simulink model "HVDC_Model"  (R2024a)
settings: Solver=VariableStepAuto  StartTime=0.0  StopTime=10.0  RelTol=1e-3
undefined symbols (not defined in the file or in its folder): D1, Delta, Fnom_I, Fnom_R, Idc_nom, lagging, pulse, Ts, Vdc_nom, VLL_nom_I, VLL_nom_R
libraries: spsThreePhaseHarmonicFilterLib x6, spsUniversalBridgeLib x4, spsGroundLib x3, spsPulseGeneratorThyristor12PulseLib x3, spsVoltageMeasurementLib x3, spsThreePhaseSourceLib x2, spsThreePhaseParallelRLCBranchLib x2, spsThreePhaseSeriesRLCLoadLib x2, spsPLL3phLib x2, spsThreePhaseTransformerThreeWindingsLib x2, spsCurrentMeasurementLib x2, spsSeriesRLCBranchLib x1
settings Model: Creator=E370_  LastModifiedBy=E370_

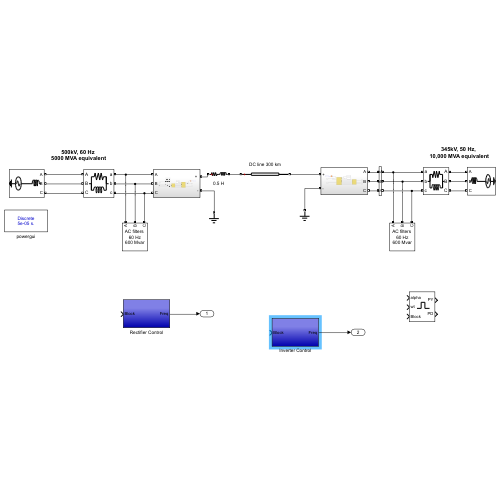
[thumbnail: Simulink's stored preview of the top-level diagram]
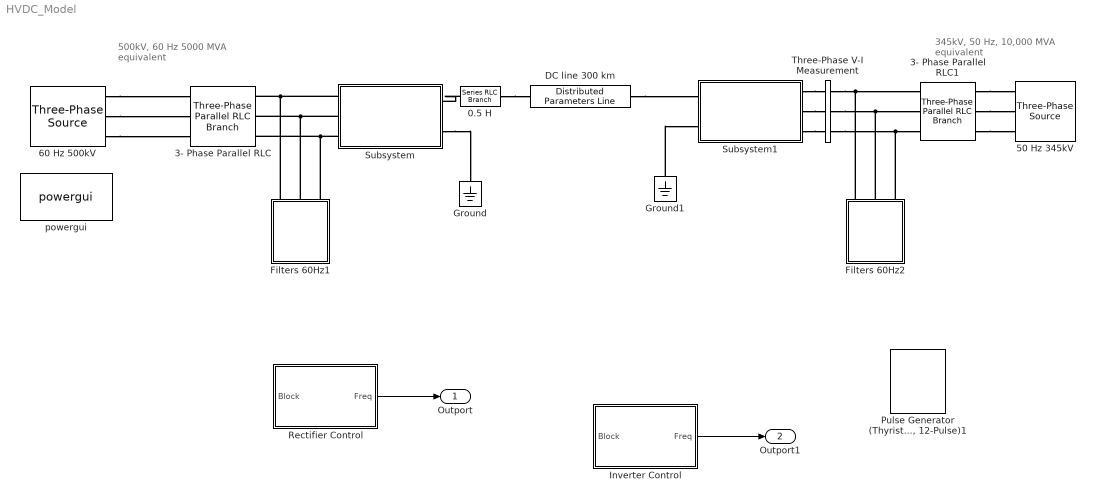
== system HVDC_Model ==
  note: 500kV, 60 Hz
      |  5000 MVA equivalent
  note: 345kV, 50 Hz,
      | 10,000 MVA equivalent
  " 50 Hz 345kV  " : spsThreePhaseSourceLib/Three-Phase Source  InternalConnection=Yg  VoltagePhases=off  Voltage=VLL_nom_I  PhaseAngle=0  Voltage_phases=[25e3 25e3 25e3]/sqrt(3)  PhaseAngles_phases=[0 -120 +120]  Frequency=Fnom_I  NonIdealSource=on  SpecifyImpedance=off  Resistance=0  Inductance=28.0e-3  ShortCircuitLevel=0  BaseVoltage=0  XRratio=0  BusType=swing  Pref=0  Qref=0  Prefabc=[10e3, 10e3, 10e3]  Qrefabc=[0, 0, 0]  Qmin=-inf  Qmax=inf
  " 60 Hz 500kV" : spsThreePhaseSourceLib/Three-Phase Source  InternalConnection=Yg  VoltagePhases=off  Voltage=VLL_nom_R  PhaseAngle=0  Voltage_phases=[25e3 25e3 25e3]/sqrt(3)  PhaseAngles_phases=[0 -120 +120]  Frequency=Fnom_R  NonIdealSource=on  SpecifyImpedance=off  Resistance=0  Inductance=98.03e-3  ShortCircuitLevel=0  BaseVoltage=0  XRratio=0  BusType=swing  Pref=0  Qref=0  Prefabc=[10e3, 10e3, 10e3]  Qrefabc=[0, 0, 0]  Qmin=-inf  Qmax=inf
  0.5 H : spsSeriesRLCBranchLib/Series RLC Branch  LConnTagsString=__new0  RConnTagsString=__new0  BranchType=RL  Resistance=1  Inductance=0.5  SetiL0=off  InitialCurrent=0  Capacitance=1.0  Setx0=off  InitialVoltage=0  Measurements=None
  3- Phase Parallel RLC : spsThreePhaseParallelRLCBranchLib/Three-Phase Parallel RLC Branch  LConnTagsString=A|B|C  RConnTagsString=A|B|C  BranchType=RL  Resistance=26.07  Inductance=48.86e-3  Capacitance=1.0  Measurements=None
  3- Phase Parallel RLC1 : spsThreePhaseParallelRLCBranchLib/Three-Phase Parallel RLC Branch  LConnTagsString=A|B|C  RConnTagsString=A|B|C  BranchType=RL  Resistance=6.205  Inductance=13.96e-3  Capacitance=1.0  Measurements=None
  DC line 300 km : spsDistributedParametersLineLib/Distributed Parameters Line  Phases=1  Length=300  Frequency=60  Resistance=0.015  Inductance=0.792e-3  Capacitance=14.4e-9  x1=[-0.00105 -6.18058111349283e-12;-0.001 -6.09272096015694e-12;-0.00095 -6.00369609044989e-12;-0.0009 -5.91353789360421e-12;-0.00085 -5.82227791484294e-12;-0.0008 -5.7299478442921e-12;-0.00075 -5.63657950590245e-12;-0.0007 -5.54220484638449e-12;-0.00065 -5.44685592416066e-12;-0.0006 -5.35056489833836e-12;-0.00055 -5.2533640177079e-12;-0.0005 -5.15528560976897e-12;-0.00045 -5.05636206978949e-12;-0.0004 -4.95662584990061e-12;-0.00035 -4.85610944823157e-12;-0.0003 -4.75484539808807e-12;-0.00025 -4.65286625717792e-12;-0.0002 -4.55020459688746e-12;-0.00015 -4.44689299161251e-12;-0.0001 -4.34296400814731e-12;-5e-05 -4.23845019513496e-12]  x2=[-0.00105 -5.4796147498648e-12;-0.001 -5.38394831103393e-12;-0.00095 -5.28731700560248e-12;-0.0009 -5.18975488737601e-12;-0.00085 -5.09129610703133e-12;-0.0008 -4.99197490010943e-12;-0.00075 -4.89182557503596e-12;-0.0007 -4.79088250117334e-12;-0.00065 -4.68918009690885e-12;-0.0006 -4.58675281778278e-12;-0.00055 -4.48363514466077e-12;-0.0005 -4.37986157195443e-12;-0.00045 -4.27546659589437e-12;-0.0004 -4.17048470285956e-12;-0.00035 -4.06495035776722e-12;-0.0003 -3.95889799252695e-12;-0.00025 -3.85236199456322e-12;-0.0002 -3.74537669541008e-12;-0.00015 -3.63797635938187e-12;-0.0001 -3.53019517232379e-12;-5e-05 -3.42206723044614e-12]  x3=[-0.00105 -3.41290835471429e-14;-0.001 -3.36568958149302e-14;-0.00095 -3.31769543764507e-14;-0.0009 -3.26894283733644e-14;-0.00085 -3.21944886050515e-14;-0.0008 -3.16923074685244e-14;-0.00075 -3.11830588980277e-14;-0.0007 -3.06669183043476e-14;-0.00065 -3.0144062513852e-14;-0.0006 -2.96146697072825e-14;-0.00055 -2.90789193583197e-14;-0.0005 -2.85369921719432e-14;-0.00045 -2.79890700226075e-14;-0.0004 -2.74353358922559e-14;-0.00035 -2.68759738081922e-14;-0.0003 -2.63111687808334e-14;-0.00025 -2.57411067413637e-14;-0.0002 -2.5165974479311e-14;-0.00015 -2.45859595800679e-14;-0.0001 -2.40012503623781e-14;-5e-05 -2.34120358158086e-14]  x4=[-0.00105 -2.27784758684538e-14;-0.001 -2.25723505250607e-14;-0.00095 -2.23621997542686e-14;-0.0009 -2.21481181558178e-14;-0.00085 -2.1930200735571e-14;-0.0008 -2.17085428670839e-14;-0.00075 -2.14832402532907e-14;-0.0007 -2.12543888883198e-14;-0.00065 -2.10220850194532e-14;-0.0006 -2.07864251092444e-14;-0.00055 -2.05475057978099e-14;-0.0005 -2.0305423865308e-14;-0.00045 -2.00602761946182e-14;-0.0004 -1.98121597342372e-14;-0.00035 -1.9561171461403e-14;-0.0003 -1.9307408345463e-14;-0.00025 -1.90509673114976e-14;-0.0002 -1.87919452042148e-14;-0.00015 -1.85304387521266e-14;-0.0001 -1.82665445320231e-14;-5e-05 -1.80003589337544e-14]  x5=0.00101312980412186  V1=ones(3,3)  V2=ones(3,3)  I1=ones(3,3)  I2=ones(3,3)  nHarmo=1  Measurements=Phase-to-ground voltages  Decoupling=off  VsMag0=0  VrMag0=0  VsAngle0=0  VrAngle0=0  IsMag0=0  IrMag0=0  IsAngle0=0  IrAngle0=0
      settings: AttributesFormatString=\n
  Filters 60Hz1 : Subsystem
      mask Display: disp('AC filters \n60 Hz\n600 Mvar')
  Filters 60Hz2 : Subsystem
      mask Display: disp('AC filters \n60 Hz\n600 Mvar')
  Ground : spsGroundLib/Ground  LConnTagsString=a
  Ground1 : spsGroundLib/Ground  LConnTagsString=a
  Inverter Control : Subsystem
  "Pulse Generator (Thyristor, 12-Pulse)1" : spsPulseGeneratorThyristor12PulseLib/Pulse Generator (Thyristor, 12-Pulse)  GenType=12-pulse  Delta=D1 (lagging)  pwidth=60  Double_Pulse=off  Ts=0
      settings: LibrarySourceBlock=|
      | sps_lib/Power Electronics/Power Electronics Control/Pulse Generator
      | (Thyristor, 12-Pulse)
  Rectifier Control : Subsystem
  Subsystem : Subsystem
  Subsystem1 : Subsystem
  Three-Phase V-I Measurement : spsThreePhaseVIMeasurementLib/Three-Phase V-I Measurement  VoltageMeasurement=phase-to-ground  SetLabelV=on  LabelV=Vabc_I  Vpu=on  VpuLL=off  CurrentMeasurement=yes  SetLabelI=on  LabelI=Iabc_I  Ipu=on  Pbase=100e6  Vbase=345e3  OutputType=Complex  PhasorSimulation=off  PSBequivalent=0
  powergui : spspowerguiLib/powergui  Priority=2  SimulationMode=Discrete  SampleTime=Ts  frequency=60  Iterations=50  frequencyindice=60  Pbase=100e6  ErrMax=1e-4  UnitsV=kV  UnitsW=MW  buscounter=0  FunctionMessages=off  echomessages=off  EnableUseOfTLC=off  CurrentSourceSwitches=off  DisableSnubberDevices=off  DisableRonSwitches=off  DisableVfSwitches=off  DisplayEquations=off  AutomaticDiscreteSolvers=off  SolverType=Tustin  Interpol=off  ExternalGateDelay=off  methode=off  Ts=0  x0status=blocks  SPID=off  SwTol=0  HookPort=off  NonlinearTolerance=1e-4  nMaxIteration=100  ContinueOnMaxIteration=off  RestoreLinks=warning  ResistiveCurrentMeasurement=off  Frange=[10:2:1500]  Ylog=off  Xlog=off  ShowGrid=off  save=off  variable=ZData  structure=0  ZoomFFT=on  StartTime=0.0  cycles=1  DisplayStyle=off  fundamental=60  FreqAxis=off  MaxFrequency=1000  frequencyindicesteady=1  RmsSteady=1  display=off
  Outport : Outport
  Outport1 : Outport  Port=2
  wires:
  Rectifier Control/1(Freq) -> Outport/1
  Inverter Control/1(Freq) -> Outport1/1
  connections:
  Subsystem/RConn2 -- Ground/LConn1
  " 60 Hz 500kV"/RConn1 -- 3- Phase Parallel RLC/LConn1
  " 60 Hz 500kV"/RConn3 -- 3- Phase Parallel RLC/LConn3
  " 60 Hz 500kV"/RConn2 -- 3- Phase Parallel RLC/LConn2
  Subsystem/LConn3 -- 3- Phase Parallel RLC/RConn3 -- Filters 60Hz1/LConn3
  Subsystem/LConn2 -- 3- Phase Parallel RLC/RConn2 -- Filters 60Hz1/LConn2
  Subsystem/LConn1 -- 3- Phase Parallel RLC/RConn1 -- Filters 60Hz1/LConn1
  3- Phase Parallel RLC1/LConn1 -- " 50 Hz 345kV  "/RConn1
  3- Phase Parallel RLC1/LConn2 -- " 50 Hz 345kV  "/RConn2
  3- Phase Parallel RLC1/LConn3 -- " 50 Hz 345kV  "/RConn3
  Filters 60Hz2/LConn1 -- 3- Phase Parallel RLC1/RConn1 -- Three-Phase V-I Measurement/RConn1
  Filters 60Hz2/LConn2 -- 3- Phase Parallel RLC1/RConn2 -- Three-Phase V-I Measurement/RConn2
  Filters 60Hz2/LConn3 -- 3- Phase Parallel RLC1/RConn3 -- Three-Phase V-I Measurement/RConn3
  0.5 H/LConn1 -- Subsystem/RConn1
  0.5 H/RConn1 -- DC line 300 km/LConn1
  DC line 300 km/RConn1 -- Subsystem1/RConn1
  Ground1/LConn1 -- Subsystem1/RConn2
  Subsystem1/LConn1 -- Three-Phase V-I Measurement/LConn1
  Subsystem1/LConn2 -- Three-Phase V-I Measurement/LConn2
  Subsystem1/LConn3 -- Three-Phase V-I Measurement/LConn3

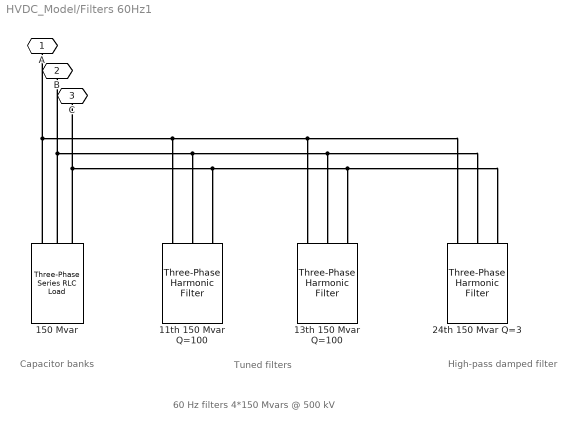
== system HVDC_Model/Filters 60Hz1 ==
  note: Capacitor banks
  note: Tuned filters
  note: High-pass
      | damped filter
  note: 60 Hz filters 4*150 Mvars @ 500 kV
  11th 150 Mvar Q=100 : spsThreePhaseHarmonicFilterLib/Three-Phase Harmonic Filter  LConnTagsString=A|B|C  FilterType=Single-tuned  FilterConnection=Y (grounded)  ParNom=[VLL_nom_R, Fnom_R]  Qc=0.25*(Vdc_nom*Idc_nom*0.6)  Fr=[11*Fnom_R]  Frd=[11*60 13*60]  Q=100  Measurements=None
      settings: AttributesFormatString=\n
  "13th 150 Mvar Q=100 " : spsThreePhaseHarmonicFilterLib/Three-Phase Harmonic Filter  LConnTagsString=A|B|C  FilterType=Single-tuned  FilterConnection=Y (grounded)  ParNom=[VLL_nom_R, Fnom_R]  Qc=0.25*(Vdc_nom*Idc_nom*0.6)  Fr=[13*Fnom_R]  Frd=[11*60 13*60]  Q=100  Measurements=None
      settings: AttributesFormatString=\n
  150 Mvar : spsThreePhaseSeriesRLCLoadLib/Three-Phase Series RLC Load  LConnTagsString=A|B|C  Configuration=Y (grounded)  NominalVoltage=VLL_nom_R  Vabc=[1e3 1e3 1e3]  Vabcp=[1e3 1e3 1e3]  NominalFrequency=Fnom_R  UnbalancedPower=off  ActivePower=0  InductivePower=0  CapacitivePower=0.25*(Vdc_nom*Idc_nom*0.6)  Pabc=[10e3 9e3 11e3]  QLabc=[100 90 110]  QCabc=[100 90 110]  Pabcp=[10e3 9e3 11e3]  QLabcp=[100 90 110]  QCabcp=[100 90 110]  Measurements=None  LoadType=constant Z
  24th 150 Mvar Q=3 : spsThreePhaseHarmonicFilterLib/Three-Phase Harmonic Filter  LConnTagsString=A|B|C  FilterType=High-pass  FilterConnection=Y (grounded)  ParNom=[VLL_nom_R, Fnom_R]  Qc=0.25*(Vdc_nom*Idc_nom*0.6)  Fr=[24*Fnom_R]  Frd=[11*60 13*60]  Q=3  Measurements=None
      settings: AttributesFormatString=\n
  A : PMIOPort  Side=Left
  B : PMIOPort  Port=2  Side=Left
  C : PMIOPort  Port=3  Side=Left
  connections:
  150 Mvar/LConn3 -- 24th 150 Mvar Q=3/LConn3 -- "13th 150 Mvar Q=100 "/LConn3 -- 11th 150 Mvar Q=100/LConn3 -- C/RConn1
  150 Mvar/LConn2 -- 24th 150 Mvar Q=3/LConn2 -- "13th 150 Mvar Q=100 "/LConn2 -- 11th 150 Mvar Q=100/LConn2 -- B/RConn1
  150 Mvar/LConn1 -- 24th 150 Mvar Q=3/LConn1 -- "13th 150 Mvar Q=100 "/LConn1 -- 11th 150 Mvar Q=100/LConn1 -- A/RConn1

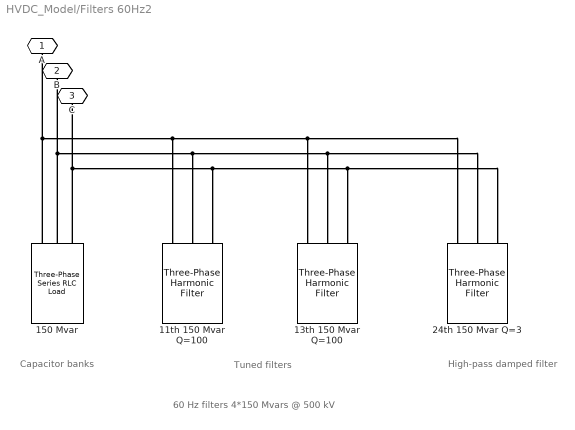
== system HVDC_Model/Filters 60Hz2 ==
  note: Capacitor banks
  note: Tuned filters
  note: High-pass
      | damped filter
  note: 60 Hz filters 4*150 Mvars @ 500 kV
  11th 150 Mvar Q=100 : spsThreePhaseHarmonicFilterLib/Three-Phase Harmonic Filter  LConnTagsString=A|B|C  FilterType=Single-tuned  FilterConnection=Y (grounded)  ParNom=[VLL_nom_R, Fnom_R]  Qc=0.25*(Vdc_nom*Idc_nom*0.6)  Fr=[11*Fnom_R]  Frd=[11*60 13*60]  Q=100  Measurements=None
      settings: AttributesFormatString=\n
  "13th 150 Mvar Q=100 " : spsThreePhaseHarmonicFilterLib/Three-Phase Harmonic Filter  LConnTagsString=A|B|C  FilterType=Single-tuned  FilterConnection=Y (grounded)  ParNom=[VLL_nom_R, Fnom_R]  Qc=0.25*(Vdc_nom*Idc_nom*0.6)  Fr=[13*Fnom_R]  Frd=[11*60 13*60]  Q=100  Measurements=None
      settings: AttributesFormatString=\n
  150 Mvar : spsThreePhaseSeriesRLCLoadLib/Three-Phase Series RLC Load  LConnTagsString=A|B|C  Configuration=Y (grounded)  NominalVoltage=VLL_nom_R  Vabc=[1e3 1e3 1e3]  Vabcp=[1e3 1e3 1e3]  NominalFrequency=Fnom_R  UnbalancedPower=off  ActivePower=0  InductivePower=0  CapacitivePower=0.25*(Vdc_nom*Idc_nom*0.6)  Pabc=[10e3 9e3 11e3]  QLabc=[100 90 110]  QCabc=[100 90 110]  Pabcp=[10e3 9e3 11e3]  QLabcp=[100 90 110]  QCabcp=[100 90 110]  Measurements=None  LoadType=constant Z
  24th 150 Mvar Q=3 : spsThreePhaseHarmonicFilterLib/Three-Phase Harmonic Filter  LConnTagsString=A|B|C  FilterType=High-pass  FilterConnection=Y (grounded)  ParNom=[VLL_nom_R, Fnom_R]  Qc=0.25*(Vdc_nom*Idc_nom*0.6)  Fr=[24*Fnom_R]  Frd=[11*60 13*60]  Q=3  Measurements=None
      settings: AttributesFormatString=\n
  A : PMIOPort  Side=Left
  B : PMIOPort  Port=2  Side=Left
  C : PMIOPort  Port=3  Side=Left
  connections:
  150 Mvar/LConn3 -- 24th 150 Mvar Q=3/LConn3 -- "13th 150 Mvar Q=100 "/LConn3 -- 11th 150 Mvar Q=100/LConn3 -- C/RConn1
  150 Mvar/LConn2 -- 24th 150 Mvar Q=3/LConn2 -- "13th 150 Mvar Q=100 "/LConn2 -- 11th 150 Mvar Q=100/LConn2 -- B/RConn1
  150 Mvar/LConn1 -- 24th 150 Mvar Q=3/LConn1 -- "13th 150 Mvar Q=100 "/LConn1 -- 11th 150 Mvar Q=100/LConn1 -- A/RConn1

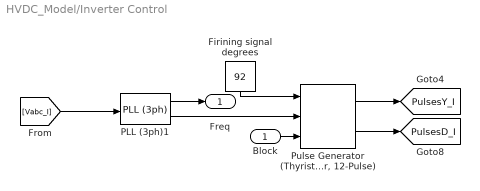
== system HVDC_Model/Inverter Control ==
  Block : Inport
  Firining signal degrees : Constant  Value=92
  PLL (3ph)1 : spsPLL3phLib/PLL (3ph)  Fmin=0.75 * 60  Par_Init=[0 60]  ParK=[180 3200 1]  TcD=1e-4  MaxRateChangeFreq=12  FilterCutOffFreq=25  Ts=Ts  AGC=off
  "Pulse Generator (Thyristor, 12-Pulse)" : spsPulseGeneratorThyristor12PulseLib/Pulse Generator (Thyristor, 12-Pulse)  GenType=12-pulse  Delta=D1 (lagging)  pwidth=60  Double_Pulse=off  Ts=0
      settings: LibrarySourceBlock=|
      | sps_lib/Power Electronics/Power Electronics Control/Pulse Generator
      | (Thyristor, 12-Pulse)
  Freq : Outport
  tag scope: PulsesD_I=global, PulsesY_I=global
  wires:
  "Pulse Generator (Thyristor, 12-Pulse)"/2 -> [PulsesD_I]
  "Pulse Generator (Thyristor, 12-Pulse)"/1 -> [PulsesY_I]
  [Vabc_I] -> PLL (3ph)1/1
  Firining signal degrees/1 -> "Pulse Generator (Thyristor, 12-Pulse)"/1
  PLL (3ph)1/2 -> "Pulse Generator (Thyristor, 12-Pulse)"/2
  Block/1 -> "Pulse Generator (Thyristor, 12-Pulse)"/3
  PLL (3ph)1/1 -> Freq/1

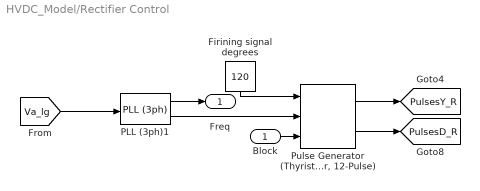
== system HVDC_Model/Rectifier Control ==
  Block : Inport
  Firining signal degrees : Constant  Value=120
  PLL (3ph)1 : spsPLL3phLib/PLL (3ph)  Fmin=0.75 * 60  Par_Init=[0 60]  ParK=[180 3200 1]  TcD=1e-4  MaxRateChangeFreq=12  FilterCutOffFreq=25  Ts=Ts  AGC=off
  "Pulse Generator (Thyristor, 12-Pulse)" : spsPulseGeneratorThyristor12PulseLib/Pulse Generator (Thyristor, 12-Pulse)  GenType=12-pulse  Delta=D1 (lagging)  pwidth=60  Double_Pulse=off  Ts=0
      settings: LibrarySourceBlock=|
      | sps_lib/Power Electronics/Power Electronics Control/Pulse Generator
      | (Thyristor, 12-Pulse)
  Freq : Outport
  tag scope: PulsesD_R=global, PulsesY_R=global
  wires:
  "Pulse Generator (Thyristor, 12-Pulse)"/2 -> [PulsesD_R]
  "Pulse Generator (Thyristor, 12-Pulse)"/1 -> [PulsesY_R]
  [Va_lg] -> PLL (3ph)1/1
  Firining signal degrees/1 -> "Pulse Generator (Thyristor, 12-Pulse)"/1
  PLL (3ph)1/2 -> "Pulse Generator (Thyristor, 12-Pulse)"/2
  Block/1 -> "Pulse Generator (Thyristor, 12-Pulse)"/3
  PLL (3ph)1/1 -> Freq/1

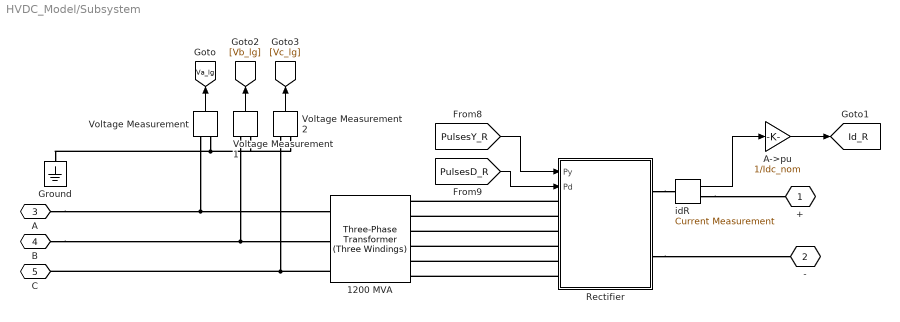
== system HVDC_Model/Subsystem ==
  1200 MVA : spsThreePhaseTransformerThreeWindingsLib/Three-Phase Transformer (Three Windings)  Winding1Connection=Yg  Winding2Connection=Y  Winding3Connection=Delta (D1)  CoreType=Three single-phase transformers  SetSaturation=off  Hysteresis=off  DataFile='hysteresis'  SetInitialFlux=off  Measurements=None  UNITS=pu  NominalPower=[ 1200e6 , 60 ]  Winding1="[VLL_nom_R*0.9 0.0025  0 ]"  Winding2=[ 200e3 0.0025 0.24]  Winding3=[ 200e3 0.0025 0.24 ]  Rm=500  Lm=500  L0=0.5  Saturation="[0 0; 0.0024 1.2; 1.0  1.45]"  InitialFluxes=[-1.26114097729929 0.657669801639854 0.603471175659435]  BreakLoop=off  DiscreteSolver=Trapezoidal iterative  DataType=off  TransfoNumber=0
      settings: AttributesFormatString=\n
  A->pu : Gain  Gain=1/Idc_nom  SaturateOnIntegerOverflow=on  OutDataTypeStr=Inherit: Same as input  ParamDataTypeStr=Inherit: Same as input
  Ground : spsGroundLib/Ground  LConnTagsString=a
  Rectifier : Subsystem
      mask Display: plot(0,0,100,100,[30 70 50 30 ], [40 40 60 40], [50 50], [25 40], [50 50], [ 60 75], [30 70], [60 60], [50 40 30], [60 70 70]);
  Voltage Measurement : spsVoltageMeasurementLib/Voltage Measurement  PhasorSimulation=off  OutputType=Complex  PSBequivalent=0
  Voltage Measurement1 : spsVoltageMeasurementLib/Voltage Measurement  PhasorSimulation=off  OutputType=Complex  PSBequivalent=0
  Voltage Measurement2 : spsVoltageMeasurementLib/Voltage Measurement  PhasorSimulation=off  OutputType=Complex  PSBequivalent=0
  idR : spsCurrentMeasurementLib/Current Measurement  Tag=PoWeRsYsTeMmEaSuReMeNt  PhasorSimulation=off  OutputType=Magnitude  PSBequivalent=0
      settings: AttributesFormatString=\n
  "+ " : PMIOPort  Side=Right
  - : PMIOPort  Port=2  Side=Right
  A : PMIOPort  Port=3  Side=Left
  B : PMIOPort  Port=4  Side=Left
  C : PMIOPort  Port=5  Side=Left
  tag scope: Id_R=global, Va_lg=global
  wires:
  idR/1 -> A->pu/1
  A->pu/1 -> [Id_R]
  [PulsesY_R] -> Rectifier/1(Py)
  [PulsesD_R] -> Rectifier/2(Pd)
  Voltage Measurement/1 -> [Va_lg]
  Voltage Measurement1/1 -> [Vb_lg]
  Voltage Measurement2/1 -> [Vc_lg]
  connections:
  Rectifier/LConn6 -- 1200 MVA/RConn6
  Rectifier/LConn5 -- 1200 MVA/RConn5
  Rectifier/LConn4 -- 1200 MVA/RConn4
  Rectifier/LConn3 -- 1200 MVA/RConn3
  Rectifier/LConn2 -- 1200 MVA/RConn2
  Rectifier/LConn1 -- 1200 MVA/RConn1
  idR/RConn1 -- "+ "/RConn1
  Rectifier/RConn2 -- -/RConn1
  Rectifier/RConn1 -- idR/LConn1
  B/RConn1 -- Voltage Measurement1/LConn1 -- 1200 MVA/LConn2
  A/RConn1 -- 1200 MVA/LConn1 -- Voltage Measurement/LConn1
  1200 MVA/LConn3 -- Voltage Measurement2/LConn1 -- C/RConn1
  Voltage Measurement/LConn2 -- Voltage Measurement2/LConn2 -- Voltage Measurement1/LConn2 -- Ground/LConn1

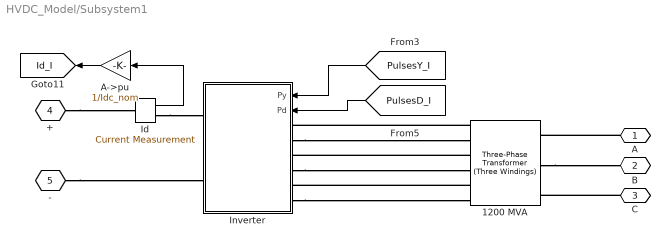
== system HVDC_Model/Subsystem1 ==
  1200 MVA : spsThreePhaseTransformerThreeWindingsLib/Three-Phase Transformer (Three Windings)  Winding1Connection=Yg  Winding2Connection=Y  Winding3Connection=Delta (D1)  CoreType=Three single-phase transformers  SetSaturation=off  Hysteresis=off  DataFile='hysteresis'  SetInitialFlux=off  Measurements=None  UNITS=pu  NominalPower=[ 1200e6 , 50 ]  Winding1="[VLL_nom_I*0.96 0.0025  0 ]"  Winding2="[ 200e3  0.0025 0.24]"  Winding3=[ 200e3 0.0025 0.24 ]  Rm=500  Lm=500  L0=0.5  Saturation="[0 0; 0.0024 1.2; 1.0  1.45]"  InitialFluxes=[-1.10749033878531 0.564800371868647 0.542689966916658]  BreakLoop=off  DiscreteSolver=Trapezoidal iterative  DataType=off  TransfoNumber=0
      settings: AttributesFormatString=\n
  A->pu : Gain  Gain=1/Idc_nom  SaturateOnIntegerOverflow=on  OutDataTypeStr=Inherit: Same as input  ParamDataTypeStr=Inherit: Same as input
  Id : spsCurrentMeasurementLib/Current Measurement  Tag=PoWeRsYsTeMmEaSuReMeNt  PhasorSimulation=off  OutputType=Magnitude  PSBequivalent=0
      settings: AttributesFormatString=\n
  Inverter : Subsystem
      mask Display: plot(0,0,100,100,[30 70 50 30 ], [60 60 40 60], [50 50], [25 40], [50 50], [ 60 75], [30 70], [40 40], [50 60 70], [40 30 30]);
  A : PMIOPort  Side=Left
  B : PMIOPort  Port=2  Side=Left
  C : PMIOPort  Port=3  Side=Left
  + : PMIOPort  Port=4  Side=Right
  - : PMIOPort  Port=5  Side=Right
  tag scope: Id_I=global
  wires:
  A->pu/1 -> [Id_I]
  Id/1 -> A->pu/1
  [PulsesY_I] -> Inverter/1(Py)
  [PulsesD_I] -> Inverter/2(Pd)
  connections:
  1200 MVA/LConn2 -- B/RConn1
  A/RConn1 -- 1200 MVA/LConn1
  +/RConn1 -- Id/LConn1
  1200 MVA/RConn3 -- Inverter/LConn3
  1200 MVA/RConn1 -- Inverter/LConn1
  C/RConn1 -- 1200 MVA/LConn3
  Inverter/LConn4 -- 1200 MVA/RConn4
  Inverter/LConn2 -- 1200 MVA/RConn2
  -/RConn1 -- Inverter/RConn2
  Id/RConn1 -- Inverter/RConn1
  1200 MVA/RConn5 -- Inverter/LConn5
  Inverter/LConn6 -- 1200 MVA/RConn6

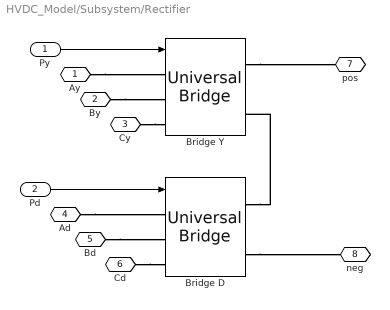
== system HVDC_Model/Subsystem/Rectifier ==
  Py : Inport
  Pd : Inport  Port=2
  Bridge D : spsUniversalBridgeLib/Universal Bridge  Arms=3  SnubberResistance=2000  SnubberCapacitance=0.1e-6  Device=Thyristors  Ron=1e-3  Lon=0  ForwardVoltages="[  0.8  0.8  ]"  ForwardVoltage=0  GTOparameters=[ 10e-6 , 20e-6 ]  IGBTparameters=[ 1e-6 , 2e-6 ]  Measurements=None  Measurements_2=None  converterType=Rectifier
      settings: AttributesFormatString=\n
  Bridge Y : spsUniversalBridgeLib/Universal Bridge  Arms=3  SnubberResistance=2000  SnubberCapacitance=0.1e-6  Device=Thyristors  Ron=1e-3  Lon=0  ForwardVoltages="[  0.8  0.8  ]"  ForwardVoltage=0  GTOparameters=[ 10e-6 , 20e-6 ]  IGBTparameters=[ 1e-6 , 2e-6 ]  Measurements=All voltages and currents  Measurements_2=None  converterType=Rectifier
      settings: AttributesFormatString=\n
  Ay : PMIOPort  Side=Left
  By : PMIOPort  Port=2  Side=Left
  Cy : PMIOPort  Port=3  Side=Left
  Ad : PMIOPort  Port=4  Side=Left
  Bd : PMIOPort  Port=5  Side=Left
  Cd : PMIOPort  Port=6  Side=Left
  pos : PMIOPort  Port=7  Side=Right
  neg : PMIOPort  Port=8  Side=Right
  wires:
  Pd/1 -> Bridge D/1
  Py/1 -> Bridge Y/1
  connections:
  Bridge D/RConn2 -- neg/RConn1
  Cd/RConn1 -- Bridge D/LConn3
  Bd/RConn1 -- Bridge D/LConn2
  Ad/RConn1 -- Bridge D/LConn1
  Cy/RConn1 -- Bridge Y/LConn3
  By/RConn1 -- Bridge Y/LConn2
  Bridge Y/RConn1 -- pos/RConn1
  Ay/RConn1 -- Bridge Y/LConn1
  Bridge D/RConn1 -- Bridge Y/RConn2

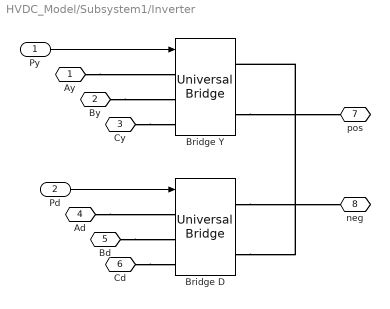
== system HVDC_Model/Subsystem1/Inverter ==
  Py : Inport
  Pd : Inport  Port=2
  Bridge D : spsUniversalBridgeLib/Universal Bridge  Arms=3  SnubberResistance=2000  SnubberCapacitance=0.1e-6  Device=Thyristors  Ron=1e-3  Lon=0  ForwardVoltages="[  0.8  0.8  ]"  ForwardVoltage=0  GTOparameters=[ 10e-6 , 20e-6 ]  IGBTparameters=[ 1e-6 , 2e-6 ]  Measurements=Device currents  Measurements_2=None  converterType=Rectifier
      settings: AttributesFormatString=\n
  Bridge Y : spsUniversalBridgeLib/Universal Bridge  Arms=3  SnubberResistance=2000  SnubberCapacitance=0.1e-6  Device=Thyristors  Ron=1e-3  Lon=0  ForwardVoltages="[  0.8  0.8  ]"  ForwardVoltage=0  GTOparameters=[ 10e-6 , 20e-6 ]  IGBTparameters=[ 1e-6 , 2e-6 ]  Measurements=All voltages and currents  Measurements_2=None  converterType=Rectifier
      settings: AttributesFormatString=\n
  Ay : PMIOPort  Side=Left
  By : PMIOPort  Port=2  Side=Left
  Cy : PMIOPort  Port=3  Side=Left
  Ad : PMIOPort  Port=4  Side=Left
  Bd : PMIOPort  Port=5  Side=Left
  Cd : PMIOPort  Port=6  Side=Left
  pos : PMIOPort  Port=7  Side=Right
  neg : PMIOPort  Port=8  Side=Right
  wires:
  Py/1 -> Bridge Y/1
  Pd/1 -> Bridge D/1
  connections:
  Bridge D/RConn1 -- neg/RConn1
  Bridge Y/RConn2 -- pos/RConn1
  Bridge D/RConn2 -- Bridge Y/RConn1
  Ay/RConn1 -- Bridge Y/LConn1
  By/RConn1 -- Bridge Y/LConn2
  Cy/RConn1 -- Bridge Y/LConn3
  Ad/RConn1 -- Bridge D/LConn1
  Bd/RConn1 -- Bridge D/LConn2
  Cd/RConn1 -- Bridge D/LConn3
